simulink model "samoletttttt"  (Simulink 7.3)
settings: Solver=ode45  StartTime=0.0  StopTime=10.0  RelTol=1e-3
libraries: simulink x1
settings Model: Creator=Sainquake Notebook  LastModifiedBy=Sainquake Notebook

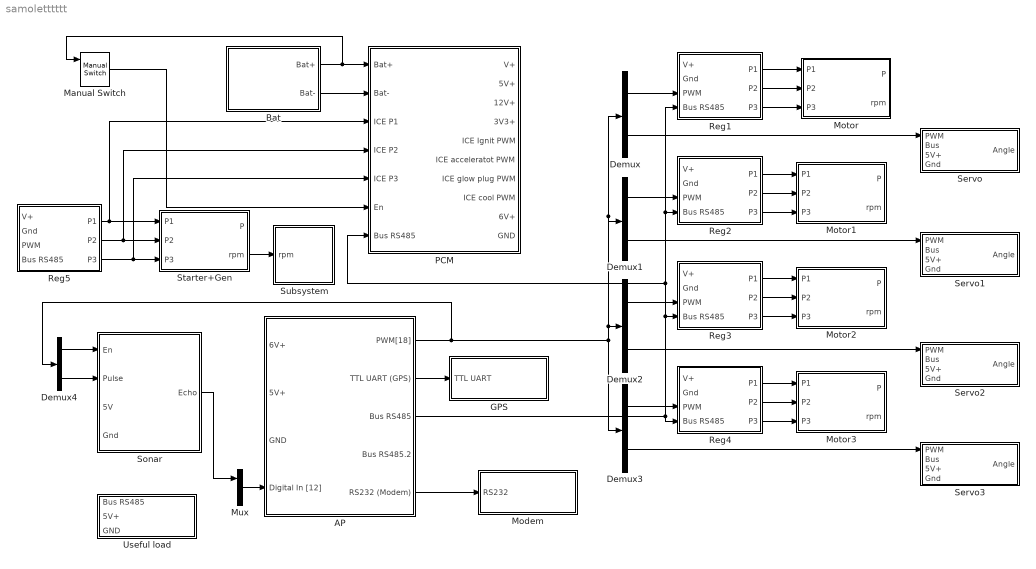
== system samoletttttt ==
  AP : Subsystem
  Bat : Subsystem
  Demux{,1..4} (5 alike) : Demux  Outputs=2
  GPS : Subsystem
  Manual Switch : simulink/Signal Routing/Manual Switch  SystemSampleTime=-1  sw=1  action=0  varsize=off
  Modem : Subsystem
  Motor : Subsystem
  Motor1 : Subsystem
  Motor2 : Subsystem
  Motor3 : Subsystem
  Mux : Mux  Inputs=2
  PCM : Subsystem
  Reg1 : Subsystem
  Reg2 : Subsystem
  Reg3 : Subsystem
  Reg4 : Subsystem
  Reg5 : Subsystem
  Servo : Subsystem
  Servo1 : Subsystem
  Servo2 : Subsystem
  Servo3 : Subsystem
  Sonar : Subsystem
  Starter+Gen : Subsystem
  Subsystem : Subsystem
  Useful load : Subsystem
  wires:
  Reg1/1(P1) -> Motor/1(P1)
  Reg1/2(P2) -> Motor/2(P2)
  Reg1/3(P3) -> Motor/3(P3)
  Reg2/1(P1) -> Motor1/1(P1)
  Reg2/2(P2) -> Motor1/2(P2)
  Reg2/3(P3) -> Motor1/3(P3)
  Reg3/1(P1) -> Motor2/1(P1)
  Reg3/2(P2) -> Motor2/2(P2)
  Reg3/3(P3) -> Motor2/3(P3)
  Reg4/1(P1) -> Motor3/1(P1)
  Reg4/2(P2) -> Motor3/2(P2)
  Reg4/3(P3) -> Motor3/3(P3)
  AP/3(Bus RS485) -> Reg4/4(Bus RS485), Reg3/4(Bus RS485), Reg2/4(Bus RS485), Reg1/4(Bus RS485), PCM/7(Bus RS485)
  Bat/1(Bat+) -> PCM/1(Bat+), Manual Switch/1
  Bat/2(Bat-) -> PCM/2(Bat-)
  Reg5/1(P1) -> Starter+Gen/1(P1), PCM/3(ICE P1)
  Reg5/2(P2) -> Starter+Gen/2(P2), PCM/4(ICE P2)
  Reg5/3(P3) -> Starter+Gen/3(P3), PCM/5(ICE P3)
  Starter+Gen/2(rpm) -> Subsystem/1(rpm)
  AP/1(PWM[18]) -> Demux3/1, Demux2/1, Demux1/1, Demux/1, Demux4/1
  AP/2(TTL UART (GPS)) -> GPS/1(TTL UART)
  AP/5(RS232 (Modem)) -> Modem/1(RS232)
  Demux3/1 -> Reg4/3(PWM)
  Demux3/2 -> Servo3/1(PWM)
  Demux2/2 -> Servo2/1(PWM)
  Demux2/1 -> Reg3/3(PWM)
  Demux1/2 -> Servo1/1(PWM)
  Demux1/1 -> Reg2/3(PWM)
  Demux/1 -> Reg1/3(PWM)
  Demux/2 -> Servo/1(PWM)
  Manual Switch/1 -> PCM/6(En)
  Demux4/1 -> Sonar/1(En)
  Demux4/2 -> Sonar/2(Pulse)
  Mux/1 -> AP/4(Digital In [12])
  Sonar/1(Echo) -> Mux/1

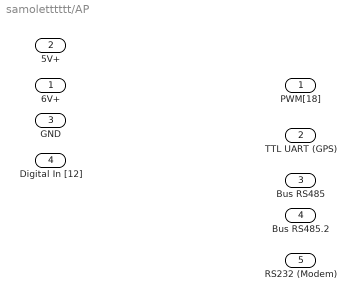
== system samoletttttt/AP ==
  6V+ : Inport  OutDataType=fixdt(1, 16)  OutScaling=2^0
  5V+ : Inport  Port=2  OutDataType=fixdt(1, 16)  OutScaling=2^0
  GND : Inport  Port=3  OutDataType=fixdt(1, 16)  OutScaling=2^0
  Digital In [12] : Inport  Port=4  OutDataType=fixdt(1, 16)  OutScaling=2^0
  PWM[18] : Outport  OutDataType=fixdt(1, 16)  OutScaling=2^0
  TTL UART (GPS) : Outport  Port=2  OutDataType=fixdt(1, 16)  OutScaling=2^0
  Bus RS485 : Outport  Port=3  OutDataType=fixdt(1, 16)  OutScaling=2^0
  Bus RS485.2 : Outport  Port=4  OutDataType=fixdt(1, 16)  OutScaling=2^0
  RS232 (Modem) : Outport  Port=5  OutDataType=fixdt(1, 16)  OutScaling=2^0

== system samoletttttt/Bat ==
  Bat+ : Outport  OutDataType=fixdt(1, 16)  OutScaling=2^0
  Bat- : Outport  Port=2  OutDataType=fixdt(1, 16)  OutScaling=2^0
  wires:
  ? -> Bat+/1

== system samoletttttt/GPS ==
  TTL UART : Inport  OutDataType=fixdt(1, 16)  OutScaling=2^0
  wires:
  TTL UART/1 -> ?

== system samoletttttt/Modem ==
  RS232 : Inport  OutDataType=fixdt(1, 16)  OutScaling=2^0
  wires:
  RS232/1 -> ?

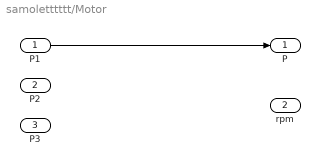
== system samoletttttt/Motor ==
  P1 : Inport  OutDataType=fixdt(1, 16)  OutScaling=2^0
  P2 : Inport  Port=2  OutDataType=fixdt(1, 16)  OutScaling=2^0
  P3 : Inport  Port=3  OutDataType=fixdt(1, 16)  OutScaling=2^0
  P : Outport  OutDataType=fixdt(1, 16)  OutScaling=2^0
  rpm : Outport  Port=2  OutDataType=fixdt(1, 16)  OutScaling=2^0
  wires:
  P1/1 -> P/1

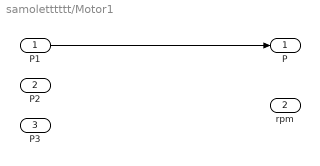
== system samoletttttt/Motor1 ==
  P1 : Inport  OutDataType=fixdt(1, 16)  OutScaling=2^0
  P2 : Inport  Port=2  OutDataType=fixdt(1, 16)  OutScaling=2^0
  P3 : Inport  Port=3  OutDataType=fixdt(1, 16)  OutScaling=2^0
  P : Outport  OutDataType=fixdt(1, 16)  OutScaling=2^0
  rpm : Outport  Port=2  OutDataType=fixdt(1, 16)  OutScaling=2^0
  wires:
  P1/1 -> P/1

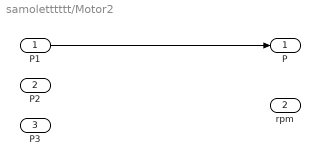
== system samoletttttt/Motor2 ==
  P1 : Inport  OutDataType=fixdt(1, 16)  OutScaling=2^0
  P2 : Inport  Port=2  OutDataType=fixdt(1, 16)  OutScaling=2^0
  P3 : Inport  Port=3  OutDataType=fixdt(1, 16)  OutScaling=2^0
  P : Outport  OutDataType=fixdt(1, 16)  OutScaling=2^0
  rpm : Outport  Port=2  OutDataType=fixdt(1, 16)  OutScaling=2^0
  wires:
  P1/1 -> P/1

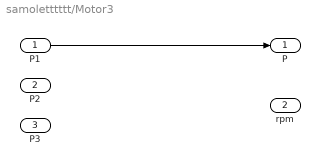
== system samoletttttt/Motor3 ==
  P1 : Inport  OutDataType=fixdt(1, 16)  OutScaling=2^0
  P2 : Inport  Port=2  OutDataType=fixdt(1, 16)  OutScaling=2^0
  P3 : Inport  Port=3  OutDataType=fixdt(1, 16)  OutScaling=2^0
  P : Outport  OutDataType=fixdt(1, 16)  OutScaling=2^0
  rpm : Outport  Port=2  OutDataType=fixdt(1, 16)  OutScaling=2^0
  wires:
  P1/1 -> P/1

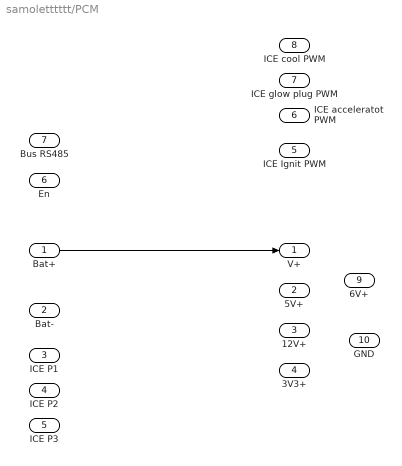
== system samoletttttt/PCM ==
  Bat+ : Inport  OutDataType=fixdt(1, 16)  OutScaling=2^0
  Bat- : Inport  Port=2  OutDataType=fixdt(1, 16)  OutScaling=2^0
  ICE P1 : Inport  Port=3  OutDataType=fixdt(1, 16)  OutScaling=2^0
  ICE P2 : Inport  Port=4  OutDataType=fixdt(1, 16)  OutScaling=2^0
  ICE P3 : Inport  Port=5  OutDataType=fixdt(1, 16)  OutScaling=2^0
  En : Inport  Port=6  OutDataType=fixdt(1, 16)  OutScaling=2^0
  Bus RS485 : Inport  Port=7  OutDataType=fixdt(1, 16)  OutScaling=2^0
  V+ : Outport  OutDataType=fixdt(1, 16)  OutScaling=2^0
  5V+ : Outport  Port=2  OutDataType=fixdt(1, 16)  OutScaling=2^0
  12V+ : Outport  Port=3  OutDataType=fixdt(1, 16)  OutScaling=2^0
  3V3+ : Outport  Port=4  OutDataType=fixdt(1, 16)  OutScaling=2^0
  ICE Ignit PWM : Outport  Port=5  OutDataType=fixdt(1, 16)  OutScaling=2^0
  "ICE acceleratot PWM " : Outport  Port=6  OutDataType=fixdt(1, 16)  OutScaling=2^0
  ICE glow plug PWM : Outport  Port=7  OutDataType=fixdt(1, 16)  OutScaling=2^0
  ICE cool PWM : Outport  Port=8  OutDataType=fixdt(1, 16)  OutScaling=2^0
  6V+ : Outport  Port=9  OutDataType=fixdt(1, 16)  OutScaling=2^0
  GND : Outport  Port=10  OutDataType=fixdt(1, 16)  OutScaling=2^0
  wires:
  Bat+/1 -> V+/1

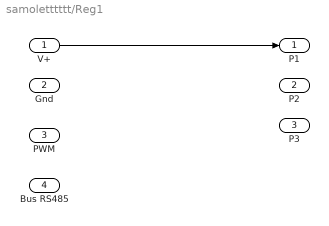
== system samoletttttt/Reg1 ==
  V+ : Inport  OutDataType=fixdt(1, 16)  OutScaling=2^0
  Gnd : Inport  Port=2  OutDataType=fixdt(1, 16)  OutScaling=2^0
  PWM : Inport  Port=3  OutDataType=fixdt(1, 16)  OutScaling=2^0
  Bus RS485 : Inport  Port=4  OutDataType=fixdt(1, 16)  OutScaling=2^0
  P1 : Outport  OutDataType=fixdt(1, 16)  OutScaling=2^0
  P2 : Outport  Port=2  OutDataType=fixdt(1, 16)  OutScaling=2^0
  P3 : Outport  Port=3  OutDataType=fixdt(1, 16)  OutScaling=2^0
  wires:
  V+/1 -> P1/1

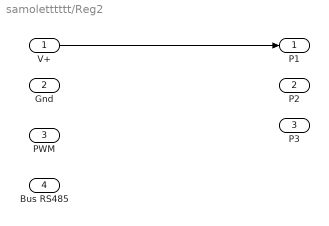
== system samoletttttt/Reg2 ==
  V+ : Inport  OutDataType=fixdt(1, 16)  OutScaling=2^0
  Gnd : Inport  Port=2  OutDataType=fixdt(1, 16)  OutScaling=2^0
  PWM : Inport  Port=3  OutDataType=fixdt(1, 16)  OutScaling=2^0
  Bus RS485 : Inport  Port=4  OutDataType=fixdt(1, 16)  OutScaling=2^0
  P1 : Outport  OutDataType=fixdt(1, 16)  OutScaling=2^0
  P2 : Outport  Port=2  OutDataType=fixdt(1, 16)  OutScaling=2^0
  P3 : Outport  Port=3  OutDataType=fixdt(1, 16)  OutScaling=2^0
  wires:
  V+/1 -> P1/1

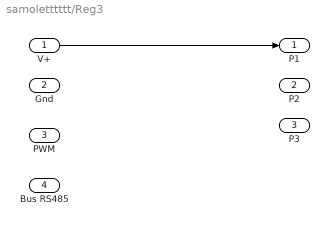
== system samoletttttt/Reg3 ==
  V+ : Inport  OutDataType=fixdt(1, 16)  OutScaling=2^0
  Gnd : Inport  Port=2  OutDataType=fixdt(1, 16)  OutScaling=2^0
  PWM : Inport  Port=3  OutDataType=fixdt(1, 16)  OutScaling=2^0
  Bus RS485 : Inport  Port=4  OutDataType=fixdt(1, 16)  OutScaling=2^0
  P1 : Outport  OutDataType=fixdt(1, 16)  OutScaling=2^0
  P2 : Outport  Port=2  OutDataType=fixdt(1, 16)  OutScaling=2^0
  P3 : Outport  Port=3  OutDataType=fixdt(1, 16)  OutScaling=2^0
  wires:
  V+/1 -> P1/1

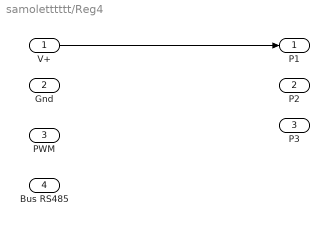
== system samoletttttt/Reg4 ==
  V+ : Inport  OutDataType=fixdt(1, 16)  OutScaling=2^0
  Gnd : Inport  Port=2  OutDataType=fixdt(1, 16)  OutScaling=2^0
  PWM : Inport  Port=3  OutDataType=fixdt(1, 16)  OutScaling=2^0
  Bus RS485 : Inport  Port=4  OutDataType=fixdt(1, 16)  OutScaling=2^0
  P1 : Outport  OutDataType=fixdt(1, 16)  OutScaling=2^0
  P2 : Outport  Port=2  OutDataType=fixdt(1, 16)  OutScaling=2^0
  P3 : Outport  Port=3  OutDataType=fixdt(1, 16)  OutScaling=2^0
  wires:
  V+/1 -> P1/1

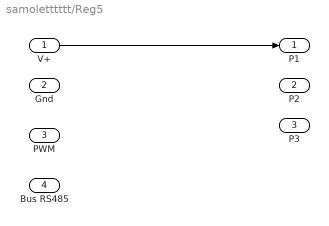
== system samoletttttt/Reg5 ==
  V+ : Inport  OutDataType=fixdt(1, 16)  OutScaling=2^0
  Gnd : Inport  Port=2  OutDataType=fixdt(1, 16)  OutScaling=2^0
  PWM : Inport  Port=3  OutDataType=fixdt(1, 16)  OutScaling=2^0
  Bus RS485 : Inport  Port=4  OutDataType=fixdt(1, 16)  OutScaling=2^0
  P1 : Outport  OutDataType=fixdt(1, 16)  OutScaling=2^0
  P2 : Outport  Port=2  OutDataType=fixdt(1, 16)  OutScaling=2^0
  P3 : Outport  Port=3  OutDataType=fixdt(1, 16)  OutScaling=2^0
  wires:
  V+/1 -> P1/1

== system samoletttttt/Servo ==
  PWM : Inport  OutDataType=fixdt(1, 16)  OutScaling=2^0
  Bus : Inport  Port=2  OutDataType=fixdt(1, 16)  OutScaling=2^0
  5V+ : Inport  Port=3  OutDataType=fixdt(1, 16)  OutScaling=2^0
  Gnd : Inport  Port=4  OutDataType=fixdt(1, 16)  OutScaling=2^0
  Angle : Outport  OutDataType=fixdt(1, 16)  OutScaling=2^0
  wires:
  PWM/1 -> Angle/1

== system samoletttttt/Servo1 ==
  PWM : Inport  OutDataType=fixdt(1, 16)  OutScaling=2^0
  Bus : Inport  Port=2  OutDataType=fixdt(1, 16)  OutScaling=2^0
  5V+ : Inport  Port=3  OutDataType=fixdt(1, 16)  OutScaling=2^0
  Gnd : Inport  Port=4  OutDataType=fixdt(1, 16)  OutScaling=2^0
  Angle : Outport  OutDataType=fixdt(1, 16)  OutScaling=2^0
  wires:
  PWM/1 -> Angle/1

== system samoletttttt/Servo2 ==
  PWM : Inport  OutDataType=fixdt(1, 16)  OutScaling=2^0
  Bus : Inport  Port=2  OutDataType=fixdt(1, 16)  OutScaling=2^0
  5V+ : Inport  Port=3  OutDataType=fixdt(1, 16)  OutScaling=2^0
  Gnd : Inport  Port=4  OutDataType=fixdt(1, 16)  OutScaling=2^0
  Angle : Outport  OutDataType=fixdt(1, 16)  OutScaling=2^0
  wires:
  PWM/1 -> Angle/1

== system samoletttttt/Servo3 ==
  PWM : Inport  OutDataType=fixdt(1, 16)  OutScaling=2^0
  Bus : Inport  Port=2  OutDataType=fixdt(1, 16)  OutScaling=2^0
  5V+ : Inport  Port=3  OutDataType=fixdt(1, 16)  OutScaling=2^0
  Gnd : Inport  Port=4  OutDataType=fixdt(1, 16)  OutScaling=2^0
  Angle : Outport  OutDataType=fixdt(1, 16)  OutScaling=2^0
  wires:
  PWM/1 -> Angle/1

== system samoletttttt/Sonar ==
  En : Inport  OutDataType=fixdt(1, 16)  OutScaling=2^0
  Pulse : Inport  Port=2  OutDataType=fixdt(1, 16)  OutScaling=2^0
  5V : Inport  Port=3  OutDataType=fixdt(1, 16)  OutScaling=2^0
  Gnd : Inport  Port=4  OutDataType=fixdt(1, 16)  OutScaling=2^0
  Echo : Outport  OutDataType=fixdt(1, 16)  OutScaling=2^0
  wires:
  En/1 -> ?

== system samoletttttt/Starter+Gen ==
  P1 : Inport  OutDataType=fixdt(1, 16)  OutScaling=2^0
  P2 : Inport  Port=2  OutDataType=fixdt(1, 16)  OutScaling=2^0
  P3 : Inport  Port=3  OutDataType=fixdt(1, 16)  OutScaling=2^0
  P : Outport  OutDataType=fixdt(1, 16)  OutScaling=2^0
  rpm : Outport  Port=2  OutDataType=fixdt(1, 16)  OutScaling=2^0
  wires:
  P1/1 -> P/1

== system samoletttttt/Subsystem ==
  rpm : Inport  OutDataType=fixdt(1, 16)  OutScaling=2^0
  wires:
  ? -> ?

== system samoletttttt/Useful load ==
  Bus RS485 : Inport  OutDataType=fixdt(1, 16)  OutScaling=2^0
  5V+ : Inport  Port=2  OutDataType=fixdt(1, 16)  OutScaling=2^0
  GND : Inport  Port=3  OutDataType=fixdt(1, 16)  OutScaling=2^0
  wires:
  Bus RS485/1 -> ?
